simulink model "gm_sampleModel1884_1_sub"  (R2023a)
settings: Solver=VariableStepAuto  StartTime=0.0  StopTime=10.0  RelTol=1e-3
libraries: simulink x2
settings Model: Creator=user1  LastModifiedBy=user1
settings OptimizationCC: BlockReduction=off  ConditionallyExecuteInputs=off
settings DebuggingCC: InheritedTsInSrcMsg=none

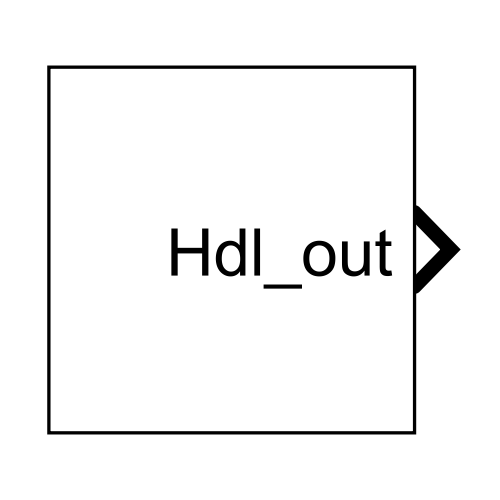
[thumbnail: Simulink's stored preview of the top-level diagram]
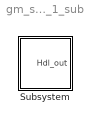
== system gm_sampleModel1884_1_sub ==
  Subsystem : Subsystem

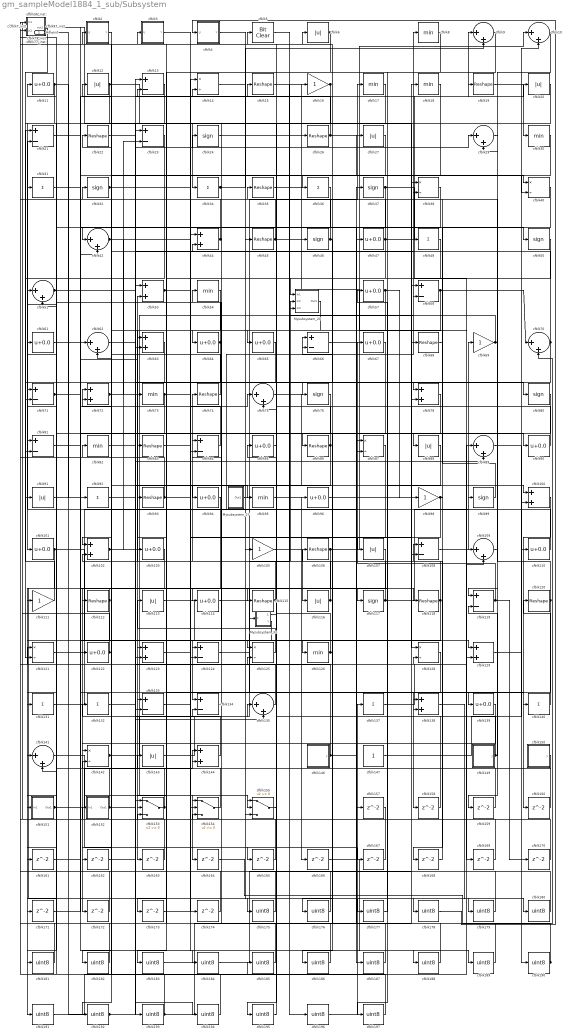
== system gm_sampleModel1884_1_sub/Subsystem ==
  Mysubsystem_20 : Subsystem
  Mysubsystem_27 : Subsystem
  Mysubsystem_33 : Subsystem
  cfblk{9..10,29,42,51,62,70,75,89,109,135,141} (12 alike) : Sum  Inputs=|++  OutDataTypeStr=uint8
  cfblk{44,53,63,72,78,100,102,123,129,138,144} (11 alike) : Sum  OutDataTypeStr=uint8
  cfblk{11,47,57,61,64..65,67,85,90,94,96,101,103,110,114,122,139} (17 alike) : Bias  Bias=0.0  SaturateOnIntegerOverflow=off
  cfblk{16,69,98,105,111} (5 alike) : Gain  OutDataTypeStr=uint8
  cfblk{15,19,22,26,35,45,68,74,83,86,93,106,112,115,118,120} (16 alike) : Reshape
  cfblk{6,12,20,27,88,91,107,113,116,143} (10 alike) : Abs  OutDataTypeStr=uint8  SaturateOnIntegerOverflow=off
  cfblk{13,21,23,58,66,71,81,84,108,119,124,133..134} (13 alike) : Sum  Inputs=+-  OutDataTypeStr=uint8
  cfblk{24,32,37,46,50,76,80,99,117} (9 alike) : Signum
  cfblk{14,38,40,87,121,125,128,142} (8 alike) : Product  Inputs=*/  OutDataTypeStr=uint8  RndMeth=Zero  SaturateOnIntegerOverflow=on
  cfblk{8,17..18,30,54,73,82,95,126} (9 alike) : MinMax  OutDataTypeStr=uint8
  cfblk127_inst : Subsystem
  cfblk{31,34,36,48,92,131..132,137,140} (9 alike) : Sum  Inputs=+  OutDataTypeStr=uint8
  cfblk136_inst : Subsystem
  cfblk146 : Subsystem  mask(Counter Limited){uplimit=double(7), tsamp=double(-1)}
      mask prompts: uplimit "Simulink:masks:UpperLimit_MP"; tsamp "Simulink:masks:SampleTime_MP"
      mask help: Simulink:masks:CounterLimited_MD
      mask init:
      | nbits = double(8);
      | tsamp = double(-1);
      | uplimit = double(7);
  cfblk147 : Constant  OutDataTypeStr=uint8  SampleTime=-1
  cfblk149 : Subsystem  mask(Counter Limited){uplimit=double(7), tsamp=double(-1)}
      mask prompts: uplimit "Simulink:masks:UpperLimit_MP"; tsamp "Simulink:masks:SampleTime_MP"
      mask help: Simulink:masks:CounterLimited_MD
      mask init:
      | nbits = double(8);
      | tsamp = double(-1);
      | uplimit = double(7);
  cfblk150 : Subsystem  mask(Counter Free-Running){NumBits=double(16), tsamp=double(-1)}
      mask prompts: NumBits "Simulink:masks:NumberOfBits_MP"; tsamp "Simulink:masks:SampleTime_MP"
      mask help: Simulink:masks:CounterFreeRunning_MD
  cfblk151 : Subsystem
  cfblk152 : Subsystem
  cfblk153 : Switch  OutDataTypeStr=uint8  SaturateOnIntegerOverflow=off  InputSameDT=off
  cfblk154 : Switch  OutDataTypeStr=uint8  SaturateOnIntegerOverflow=off  InputSameDT=off
  cfblk155 : Switch  OutDataTypeStr=uint8  SaturateOnIntegerOverflow=off  InputSameDT=off
  cfblk{157..174} (18 alike) : Delay  SampleTime=1
  cfblk{175..197} (23 alike) : DataTypeConversion  OutDataTypeStr=uint8  SaturateOnIntegerOverflow=off  RndMeth=Floor
  cfblk2 : Subsystem  mask(Detect Fall Nonpositive){vinit=double(0), InputProcessing=Elements as channels (sample based), OutDataTypeStr=uint8}
      mask prompts: vinit "Simulink:masks:InitialCondition_MP"; InputProcessing "Simulink:masks:InputProcessing_MP"; OutDataTypeStr "Simulink:masks:OutputDataType_MP"
      mask help: Simulink:masks:DetectFallNonpositive_MD
      mask init:
      | InputProcessing = 'Elements as channels (sample based)';
      | OutDataTypeStr = 'uint8';
      | vinit = double(0);
      mask TypeOptions InputProcessing: Simulink:masks:ColumnsAsChannelsFrameBased | Simulink:masks:ElementsAsChannelsSampleBased
      mask TypeOptions OutDataTypeStr: Simulink:masks:uint8 | Simulink:masks:boolean
      mask Display: fprintf('U <= 0\n&  NOT\nU/z <= 0')
  cfblk25_inst : Subsystem
  cfblk3 : Subsystem  mask(Detect Rise Positive){vinit=double(0), InputProcessing=Elements as channels (sample based), OutDataTypeStr=uint8}
      mask prompts: vinit "Simulink:masks:InitialCondition_MP"; InputProcessing "Simulink:masks:InputProcessing_MP"; OutDataTypeStr "Simulink:masks:OutputDataType_MP"
      mask help: Simulink:masks:DetectRisePositive_MD
      mask init:
      | InputProcessing = 'Elements as channels (sample based)';
      | OutDataTypeStr = 'uint8';
      | vinit = double(0);
      mask TypeOptions InputProcessing: Simulink:masks:ColumnsAsChannelsFrameBased | Simulink:masks:ElementsAsChannelsSampleBased
      mask TypeOptions OutDataTypeStr: Simulink:masks:uint8 | Simulink:masks:boolean
      mask Display: fprintf('U > 0\n&  NOT\nU/z > 0')
  cfblk4 : Subsystem  mask(Detect Rise Positive){vinit=double(0), InputProcessing=Elements as channels (sample based), OutDataTypeStr=uint8}
      mask prompts: vinit "Simulink:masks:InitialCondition_MP"; InputProcessing "Simulink:masks:InputProcessing_MP"; OutDataTypeStr "Simulink:masks:OutputDataType_MP"
      mask help: Simulink:masks:DetectRisePositive_MD
      mask init:
      | InputProcessing = 'Elements as channels (sample based)';
      | OutDataTypeStr = 'uint8';
      | vinit = double(0);
      mask TypeOptions InputProcessing: Simulink:masks:ColumnsAsChannelsFrameBased | Simulink:masks:ElementsAsChannelsSampleBased
      mask TypeOptions OutDataTypeStr: Simulink:masks:uint8 | Simulink:masks:boolean
      mask Display: fprintf('U > 0\n&  NOT\nU/z > 0')
  cfblk49_inst : Subsystem
  cfblk5 : simulink/Logic and Bit Operations/Bit Clear  iBit=0
      settings: LibrarySourceBlock=|
      | hdlsllib/Logic and Bit
      | Operations/Bit Clear
  cfblk52_inst : Subsystem
  cfblk56_inst : Subsystem
  cfblk77_inst : Subsystem
  cfblk79_inst : Subsystem
  cfblk7_inst : Subsystem
  cfblk97_inst : Subsystem
  Hdl_out : Outport  OutDataTypeStr=uint8  SampleTime=1
  wires:
  Mysubsystem_20/1(Out1) -> cfblk163/1
  Mysubsystem_27/1(Out1) -> cfblk100/1
  Mysubsystem_33/1(Out1) -> cfblk8/1
  Mysubsystem_33/2(Y) -> cfblk141/2
  cfblk10/1 -> cfblk29/2
  cfblk100/1 -> cfblk160/1
  cfblk101/1 -> cfblk178/1, cfblk129/1
  cfblk102/1 -> cfblk58/2, cfblk23/2, cfblk155/2
  cfblk103/1 -> cfblk191/1
  cfblk105/1 -> cfblk116/1
  cfblk106/1 -> cfblk10/1, cfblk172/1
  cfblk107/1 -> cfblk133/1
  cfblk108/1 -> cfblk69/1
  cfblk109/1 -> cfblk159/1
  cfblk11/1 -> cfblk101/1, cfblk92/1
  cfblk110/1 -> cfblk21/2
  cfblk111/1 -> cfblk21/1
  cfblk112/1 -> cfblk141/1, cfblk111/1
  cfblk113/1 -> cfblk126/1
  cfblk114/1 -> cfblk140/1
  cfblk115/1 -> cfblk53/2, cfblk22/1
  cfblk116/1 -> cfblk23/1, Mysubsystem_20/2(In2)
  cfblk117/1 -> cfblk99/1, cfblk74/1
  cfblk118/1 -> cfblk53/1, cfblk134/1, cfblk106/1
  cfblk119/1 -> cfblk67/1, cfblk170/1
  cfblk12/1 -> cfblk161/1, cfblk34/1
  cfblk120/1 -> cfblk35/1, cfblk158/1
  cfblk121/1 -> cfblk87/1
  cfblk122/1 -> cfblk62/2, cfblk49_inst/1(in1)
  cfblk123/1 -> cfblk174/1
  cfblk124/1 -> cfblk17/1
  cfblk125/1 -> cfblk113/1
  cfblk126/1 -> cfblk6/1, cfblk31/1
  cfblk127_inst/1(out1) -> cfblk128/1
  cfblk128/1 -> cfblk153/2
  cfblk129/1 -> cfblk10/2
  cfblk13/1 -> cfblk131/1
  cfblk131/1 -> cfblk16/1
  cfblk132/1 -> cfblk193/1
  cfblk133/1 -> cfblk27/1
  cfblk134/1 -> cfblk54/1
  cfblk135/1 -> cfblk77_inst/1(in1)
  cfblk136_inst/1(out1) -> cfblk105/1
  cfblk137/1 -> cfblk109/1
  cfblk138/1 -> cfblk180/1
  cfblk139/1 -> cfblk142/1
  cfblk14/1 -> cfblk45/1
  cfblk140/1 -> cfblk120/1
  cfblk141/1 -> cfblk165/1
  cfblk142/1 -> cfblk134/2, cfblk164/1
  cfblk143/1 -> cfblk46/1
  cfblk144/1 -> cfblk12/1
  cfblk146/1(y) -> cfblk47/1, cfblk82/1
  cfblk147/1 -> cfblk110/1
  cfblk149/1(y) -> cfblk119/2, cfblk14/2
  cfblk15/1 -> cfblk169/1
  cfblk150/1(y) -> cfblk142/2
  cfblk151/1(Out1) -> cfblk154/1, cfblk144/1, cfblk121/1
  cfblk152/1(Out1) -> cfblk135/1, cfblk127_inst/1(in1)
  cfblk153/1 -> cfblk72/1, cfblk32/1
  cfblk154/1 -> cfblk2/1(U)
  cfblk155/1 -> cfblk85/1
  cfblk157/1 -> cfblk153/3
  cfblk158/1 -> cfblk44/2
  cfblk159/1 -> cfblk71/1
  cfblk16/1 -> cfblk65/1, cfblk121/2
  cfblk160/1 -> cfblk84/1
  cfblk161/1 -> cfblk42/2
  cfblk162/1 -> cfblk128/2
  cfblk163/1 -> cfblk136_inst/2(in2)
  cfblk164/1 -> cfblk70/2
  cfblk165/1 -> cfblk52_inst/1(in1)
  cfblk166/1 -> cfblk189/1
  cfblk167/1 -> cfblk153/1
  cfblk168/1 -> cfblk108/1
  cfblk169/1 -> cfblk58/1
  cfblk17/1 -> cfblk114/1
  cfblk170/1 -> cfblk102/2
  cfblk171/1 -> cfblk63/1
  cfblk172/1 -> cfblk51/1
  cfblk173/1 -> cfblk125/2
  cfblk174/1 -> cfblk81/1
  cfblk175/1 -> cfblk11/1
  cfblk176/1 -> cfblk3/1(U)
  cfblk177/1 -> cfblk57/1
  cfblk178/1 -> cfblk4/1(U)
  cfblk179/1 -> cfblk75/2
  cfblk18/1 -> cfblk182/1
  cfblk180/1 -> cfblk25_inst/1(in1)
  cfblk181/1 -> cfblk25_inst/2(in2)
  cfblk182/1 -> cfblk79_inst/1(in1)
  cfblk183/1 -> cfblk18/1
  cfblk184/1 -> cfblk68/1
  cfblk185/1 -> cfblk7_inst/1(in1)
  cfblk186/1 -> cfblk7_inst/2(in2)
  cfblk187/1 -> cfblk143/1
  cfblk188/1 -> cfblk66/1
  cfblk189/1 -> cfblk66/2
  cfblk19/1 -> cfblk30/1
  cfblk190/1 -> cfblk72/2, cfblk154/3, cfblk144/2, cfblk152/1(In1)
  cfblk191/1 -> cfblk89/1
  cfblk192/1 -> cfblk89/2, Hdl_out/1
  cfblk193/1 -> cfblk79_inst/2(in2), cfblk37/1, cfblk185/1
  cfblk194/1 -> cfblk132/1
  cfblk195/1 -> cfblk5/1
  cfblk196/1 -> cfblk137/1
  cfblk197/1 -> cfblk61/1
  cfblk2/1(Y) -> cfblk162/1
  cfblk20/1 -> cfblk63/2
  cfblk21/1 -> cfblk40/1
  cfblk22/1 -> cfblk95/1
  cfblk23/1 -> cfblk71/2
  cfblk24/1 -> cfblk26/1
  cfblk25_inst/1(out1) -> cfblk179/1
  cfblk26/1 -> cfblk15/1, cfblk40/2
  cfblk27/1 -> cfblk36/1
  cfblk29/1 -> cfblk139/1
  cfblk3/1(Y) -> cfblk175/1
  cfblk30/1 -> cfblk42/1
  cfblk31/1 -> cfblk86/1
  cfblk32/1 -> cfblk155/1, cfblk108/2
  cfblk34/1 -> cfblk9/2, cfblk155/3, cfblk124/1
  cfblk35/1 -> cfblk157/1
  cfblk36/1 -> Mysubsystem_33/1(In1)
  cfblk37/1 -> cfblk109/2, cfblk87/2
  cfblk38/1 -> cfblk171/1
  cfblk4/1(Y) -> cfblk177/1
  cfblk40/1 -> cfblk78/1
  cfblk42/1 -> cfblk80/1, cfblk73/1
  cfblk44/1 -> cfblk64/1, cfblk136_inst/1(in1)
  cfblk45/1 -> cfblk96/1, cfblk127_inst/2(in2)
  cfblk46/1 -> cfblk76/1, cfblk49_inst/2(in2)
  cfblk47/1 -> cfblk9/1, cfblk123/1, cfblk14/1
  cfblk48/1 -> cfblk94/1
  cfblk49_inst/1(out1) -> cfblk50/1, cfblk118/1
  cfblk5/1 -> cfblk196/1
  cfblk50/1 -> Mysubsystem_20/1(In1)
  cfblk51/1 -> cfblk19/1, cfblk135/2
  cfblk52_inst/1(out1) -> cfblk84/2
  cfblk53/1 -> cfblk129/2, cfblk167/1
  cfblk54/1 -> cfblk112/1
  cfblk56_inst/1(out1) -> cfblk91/1
  cfblk57/1 -> cfblk115/1, cfblk98/1
  cfblk58/1 -> cfblk93/1, cfblk70/1
  cfblk6/1 -> cfblk77_inst/2(in2), cfblk124/2
  cfblk61/1 -> cfblk62/1
  cfblk62/1 -> cfblk20/1
  cfblk63/1 -> cfblk81/2
  cfblk64/1 -> cfblk97_inst/2(in2), cfblk192/1
  cfblk65/1 -> cfblk173/1
  cfblk66/1 -> cfblk187/1
  cfblk67/1 -> cfblk176/1
  cfblk68/1 -> cfblk138/2
  cfblk69/1 -> cfblk119/1, Mysubsystem_20/3(In3)
  cfblk7_inst/1(out1) -> cfblk184/1
  cfblk70/1 -> cfblk52_inst/2(in2), cfblk123/2
  cfblk71/1 -> cfblk51/2, cfblk13/2
  cfblk72/1 -> cfblk78/2, cfblk194/1
  cfblk73/1 -> cfblk83/1, cfblk188/1
  cfblk74/1 -> cfblk56_inst/2(in2)
  cfblk75/1 -> cfblk100/2
  cfblk76/1 -> cfblk103/1
  cfblk77_inst/1(out1) -> cfblk88/1
  cfblk78/1 -> cfblk151/1(In1)
  cfblk79_inst/1(out1) -> cfblk138/1
  cfblk8/1 -> cfblk197/1
  cfblk80/1 -> cfblk181/1
  cfblk81/1 -> cfblk125/1
  cfblk82/1 -> cfblk48/1
  cfblk83/1 -> cfblk90/1
  cfblk84/1 -> cfblk44/1
  cfblk85/1 -> cfblk195/1
  cfblk86/1 -> cfblk13/1, cfblk102/1
  cfblk87/1 -> cfblk107/1
  cfblk88/1 -> cfblk117/1
  cfblk89/1 -> cfblk190/1
  cfblk9/1 -> cfblk183/1
  cfblk90/1 -> cfblk56_inst/1(in1)
  cfblk91/1 -> cfblk75/1
  cfblk92/1 -> cfblk24/1
  cfblk93/1 -> cfblk97_inst/1(in1), cfblk29/1
  cfblk94/1 -> cfblk122/1
  cfblk95/1 -> cfblk166/1
  cfblk96/1 -> cfblk38/1
  cfblk97_inst/1(out1) -> cfblk133/2
  cfblk98/1 -> cfblk186/1, cfblk154/2, cfblk168/1
  cfblk99/1 -> cfblk38/2

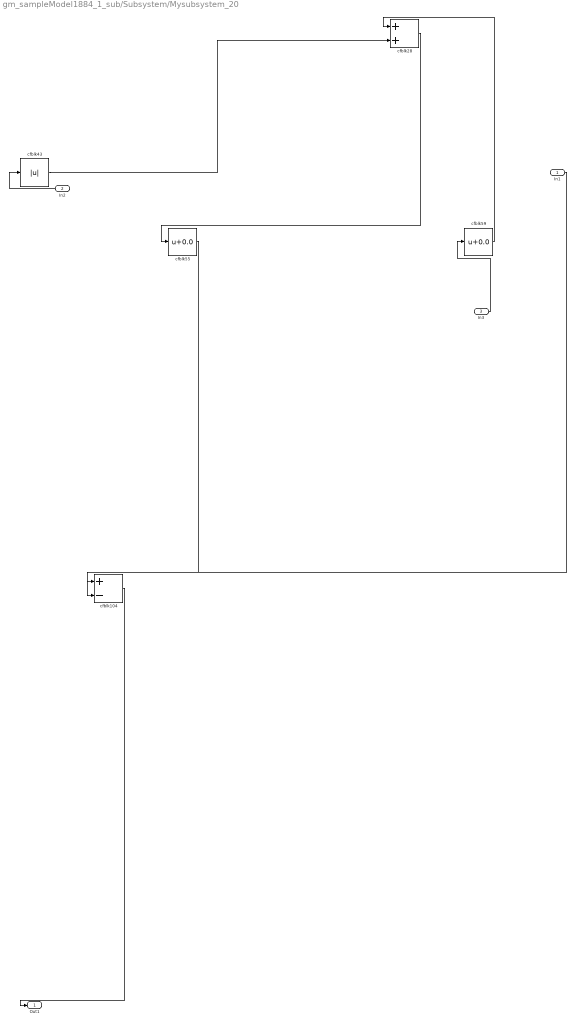
== system gm_sampleModel1884_1_sub/Subsystem/Mysubsystem_20 ==
  In1 : Inport  OutDataTypeStr=uint8  PortDimensions=1  SampleTime=1
  In2 : Inport  Port=2  OutDataTypeStr=uint8  PortDimensions=1  SampleTime=1
  In3 : Inport  Port=3  OutDataTypeStr=uint8  PortDimensions=1  SampleTime=1
  cfblk104 : Sum  Inputs=+-
  cfblk28 : Sum
  cfblk43 : Abs  SaturateOnIntegerOverflow=off
  cfblk55 : Bias  Bias=0.0  SaturateOnIntegerOverflow=off
  cfblk59 : Bias  Bias=0.0  SaturateOnIntegerOverflow=off
  Out1 : Outport  SampleTime=1
  wires:
  In1/1 -> cfblk104/2
  In2/1 -> cfblk43/1
  In3/1 -> cfblk59/1
  cfblk104/1 -> Out1/1
  cfblk28/1 -> cfblk55/1
  cfblk43/1 -> cfblk28/2
  cfblk55/1 -> cfblk104/1
  cfblk59/1 -> cfblk28/1

== system gm_sampleModel1884_1_sub/Subsystem/Mysubsystem_27 ==
  cfblk148 : Ground
  cfblk41 : Sum  Inputs=+
  Out1 : Outport  SampleTime=1
  wires:
  cfblk148/1 -> cfblk41/1
  cfblk41/1 -> Out1/1

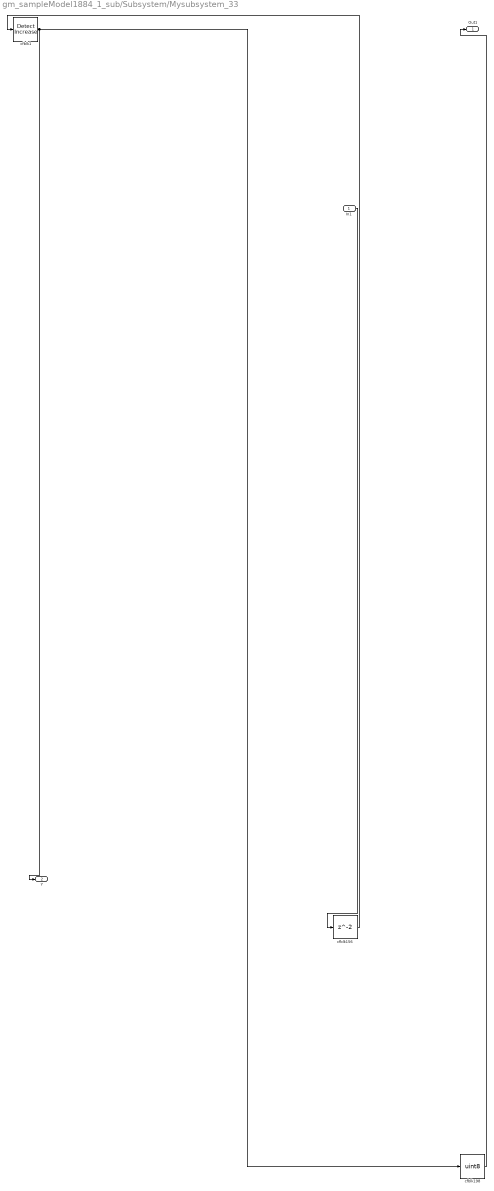
== system gm_sampleModel1884_1_sub/Subsystem/Mysubsystem_33 ==
  In1 : Inport  OutDataTypeStr=uint8  PortDimensions=1  SampleTime=1
  cfblk1 : simulink/Logic and Bit Operations/Detect Increase  vinit=0.0  OutDataTypeStr=boolean
      settings: LibrarySourceBlock=|
      | hdlsllib/Logic and Bit
      | Operations/Detect
      | Increase
  cfblk156 : Delay  SampleTime=1
  cfblk198 : DataTypeConversion  OutDataTypeStr=uint8  SaturateOnIntegerOverflow=off  RndMeth=Floor
  Out1 : Outport  SampleTime=1
  Y : Outport  Port=2  SampleTime=1
  wires:
  In1/1 -> cfblk156/1
  cfblk1/1 -> cfblk198/1, Y/1
  cfblk156/1 -> cfblk1/1
  cfblk198/1 -> Out1/1

== system gm_sampleModel1884_1_sub/Subsystem/cfblk127_inst ==
  in1 : Inport  OutDataTypeStr=uint8  SampleTime=1
  in2 : Inport  Port=2  OutDataTypeStr=uint8  SampleTime=1
  mul_cfblk127_dotp_mulcomp : Product  Inputs=**  OutDataTypeStr=uint8  SampleTime=1
  out1 : Outport  OutDataTypeStr=uint8  SampleTime=1
  wires:
  in1/1 -> mul_cfblk127_dotp_mulcomp/1
  in2/1 -> mul_cfblk127_dotp_mulcomp/2
  mul_cfblk127_dotp_mulcomp/1 -> out1/1

== system gm_sampleModel1884_1_sub/Subsystem/cfblk136_inst ==
  in1 : Inport  OutDataTypeStr=uint8  SampleTime=1
  in2 : Inport  Port=2  OutDataTypeStr=uint8  SampleTime=1
  mul_cfblk136_dotp_mulcomp : Product  Inputs=**  OutDataTypeStr=uint8  SampleTime=1
  out1 : Outport  OutDataTypeStr=uint8  SampleTime=1
  wires:
  in1/1 -> mul_cfblk136_dotp_mulcomp/1
  in2/1 -> mul_cfblk136_dotp_mulcomp/2
  mul_cfblk136_dotp_mulcomp/1 -> out1/1

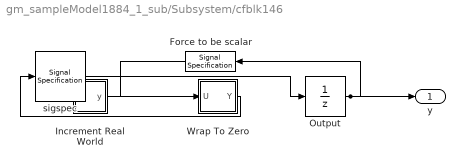
== system gm_sampleModel1884_1_sub/Subsystem/cfblk146 ==
  Force to be scalar : SignalSpecification  DisableCoverage=on  Dimensions=1
  Increment Real World : Subsystem  mask(Real World Value Increment){}
      mask help: Simulink:masks:RealWorldValueIncrement_MD
      mask Display: disp('V++')
  Output : UnitDelay  InitialCondition=0.0  SampleTime=tsamp  HasFrameUpgradeWarning=on
  Wrap To Zero : Subsystem  mask(Wrap To Zero){Threshold=double(7)}
      mask prompts: Threshold "Simulink:masks:Threshold_MP"
      mask help: Simulink:masks:WrapToZero_MD
  sigspec : SignalSpecification  OutDataTypeStr=uint8  Dimensions=1
  y : Outport  SampleTime=1
  wires:
  Force to be scalar/1 -> Increment Real World/1(u)
  Increment Real World/1(y) -> Wrap To Zero/1(U)
  Output/1 -> Force to be scalar/1, y/1
  Wrap To Zero/1(Y) -> sigspec/1
  sigspec/1 -> Output/1

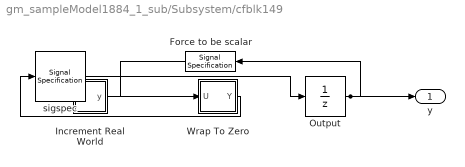
== system gm_sampleModel1884_1_sub/Subsystem/cfblk149 ==
  Force to be scalar : SignalSpecification  DisableCoverage=on  Dimensions=1
  Increment Real World : Subsystem  mask(Real World Value Increment){}
      mask help: Simulink:masks:RealWorldValueIncrement_MD
      mask Display: disp('V++')
  Output : UnitDelay  InitialCondition=0.0  SampleTime=tsamp  HasFrameUpgradeWarning=on
  Wrap To Zero : Subsystem  mask(Wrap To Zero){Threshold=double(7)}
      mask prompts: Threshold "Simulink:masks:Threshold_MP"
      mask help: Simulink:masks:WrapToZero_MD
  sigspec : SignalSpecification  OutDataTypeStr=uint8  Dimensions=1
  y : Outport  SampleTime=1
  wires:
  Force to be scalar/1 -> Increment Real World/1(u)
  Increment Real World/1(y) -> Wrap To Zero/1(U)
  Output/1 -> Force to be scalar/1, y/1
  Wrap To Zero/1(Y) -> sigspec/1
  sigspec/1 -> Output/1

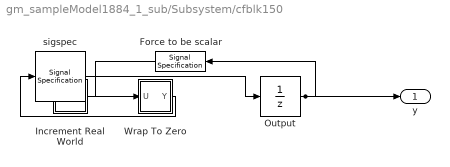
== system gm_sampleModel1884_1_sub/Subsystem/cfblk150 ==
  Force to be scalar : SignalSpecification  DisableCoverage=on  Dimensions=1
  Increment Real World : Subsystem  mask(Real World Value Increment){}
      mask help: Simulink:masks:RealWorldValueIncrement_MD
      mask Display: disp('V++')
  Output : UnitDelay  InitialCondition=0.0  SampleTime=tsamp  HasFrameUpgradeWarning=on
  Wrap To Zero : Subsystem  mask(Wrap To Zero){Threshold=double(65535)}
      mask prompts: Threshold "Simulink:masks:Threshold_MP"
      mask help: Simulink:masks:WrapToZero_MD
  sigspec : SignalSpecification  OutDataTypeStr=uint16  Dimensions=1
  y : Outport  SampleTime=1
  wires:
  Force to be scalar/1 -> Increment Real World/1(u)
  Increment Real World/1(y) -> Wrap To Zero/1(U)
  Output/1 -> Force to be scalar/1, y/1
  Wrap To Zero/1(Y) -> sigspec/1
  sigspec/1 -> Output/1

== system gm_sampleModel1884_1_sub/Subsystem/cfblk151 ==
  In1 : Inport  OutDataTypeStr=uint8  PortDimensions=1  SampleTime=1
  Out1 : Outport  SampleTime=1
  wires:
  In1/1 -> Out1/1

== system gm_sampleModel1884_1_sub/Subsystem/cfblk152 ==
  In1 : Inport  OutDataTypeStr=uint8  PortDimensions=1  SampleTime=1
  Out1 : Outport  SampleTime=1
  wires:
  In1/1 -> Out1/1

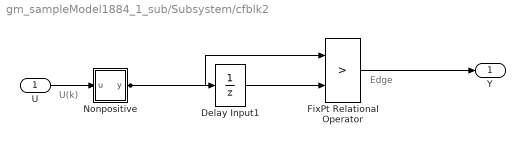
== system gm_sampleModel1884_1_sub/Subsystem/cfblk2 ==
  note: U(k)
  note: Edge
  U : Inport  OutDataTypeStr=uint8  SampleTime=1
  Delay Input1 : UnitDelay  Description=Store in Global RAM  DisableCoverage=on  InitialCondition=vinit  SampleTime=-1  HasFrameUpgradeWarning=on
  FixPt Relational Operator : RelationalOperator  Operator=>  OutDataTypeStr=fixdt(0, 8)  ZeroCross=off  InputSameDT=off
  Nonpositive : Subsystem  mask(Compare To Zero){relop=<=, OutDataTypeStr=boolean, ZeroCross=off}
      mask prompts: relop "Simulink:masks:Operator_MP"; OutDataTypeStr "Simulink:masks:OutputDataType_MP"; ZeroCross "Simulink:masks:EnableZerocrossingDetection_MP"
      mask help: Simulink:masks:CompareToZero_MD
      mask init:
      | OutDataTypeStr = 'boolean';
      | ZeroCross = 'off';
      | blkName = 'sampleModel1884_1_sub/Subsystem/cfblk2/Nonpositive';
      | relop = '<=';
      | setValue = 'boolean';
      mask TypeOptions relop: == | ~= | < | <= | >= | >
      mask TypeOptions OutDataTypeStr: Simulink:masks:uint8 | Simulink:masks:boolean
      mask Callback ZeroCross: sl('zeroCrossEnable', gcbh);
      mask Display: disp([relop,' 0'])
  Y : Outport  SampleTime=1
  wires:
  U/1 -> Nonpositive/1(u)
  Delay Input1/1 -> FixPt Relational Operator/2
  FixPt Relational Operator/1 -> Y/1
  Nonpositive/1(y) -> FixPt Relational Operator/1, Delay Input1/1

== system gm_sampleModel1884_1_sub/Subsystem/cfblk25_inst ==
  in1 : Inport  OutDataTypeStr=uint8  SampleTime=1
  in2 : Inport  Port=2  OutDataTypeStr=uint8  SampleTime=1
  mul_cfblk25_dotp_mulcomp : Product  Inputs=**  OutDataTypeStr=uint8  SampleTime=1
  out1 : Outport  OutDataTypeStr=uint8  SampleTime=1
  wires:
  in1/1 -> mul_cfblk25_dotp_mulcomp/1
  in2/1 -> mul_cfblk25_dotp_mulcomp/2
  mul_cfblk25_dotp_mulcomp/1 -> out1/1

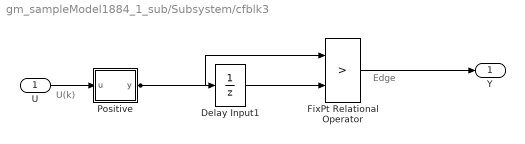
== system gm_sampleModel1884_1_sub/Subsystem/cfblk3 ==
  note: U(k)
  note: Edge
  U : Inport  OutDataTypeStr=uint8  SampleTime=1
  Delay Input1 : UnitDelay  Description=Store in Global RAM  DisableCoverage=on  InitialCondition=vinit  SampleTime=-1  HasFrameUpgradeWarning=on
  FixPt Relational Operator : RelationalOperator  Operator=>  OutDataTypeStr=fixdt(0, 8)  ZeroCross=off  InputSameDT=off
  Positive : Subsystem  mask(Compare To Zero){relop=>, OutDataTypeStr=boolean, ZeroCross=off}
      mask prompts: relop "Simulink:masks:Operator_MP"; OutDataTypeStr "Simulink:masks:OutputDataType_MP"; ZeroCross "Simulink:masks:EnableZerocrossingDetection_MP"
      mask help: Simulink:masks:CompareToZero_MD
      mask init:
      | OutDataTypeStr = 'boolean';
      | ZeroCross = 'off';
      | blkName = 'sampleModel1884_1_sub/Subsystem/cfblk3/Positive';
      | relop = '>';
      | setValue = 'boolean';
      mask TypeOptions relop: == | ~= | < | <= | >= | >
      mask TypeOptions OutDataTypeStr: Simulink:masks:uint8 | Simulink:masks:boolean
      mask Callback ZeroCross: sl('zeroCrossEnable', gcbh);
      mask Display: disp([relop,' 0'])
  Y : Outport  SampleTime=1
  wires:
  U/1 -> Positive/1(u)
  Delay Input1/1 -> FixPt Relational Operator/2
  FixPt Relational Operator/1 -> Y/1
  Positive/1(y) -> FixPt Relational Operator/1, Delay Input1/1

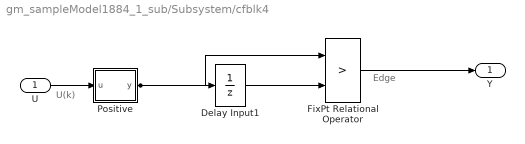
== system gm_sampleModel1884_1_sub/Subsystem/cfblk4 ==
  note: U(k)
  note: Edge
  U : Inport  OutDataTypeStr=uint8  SampleTime=1
  Delay Input1 : UnitDelay  Description=Store in Global RAM  DisableCoverage=on  InitialCondition=vinit  SampleTime=-1  HasFrameUpgradeWarning=on
  FixPt Relational Operator : RelationalOperator  Operator=>  OutDataTypeStr=fixdt(0, 8)  ZeroCross=off  InputSameDT=off
  Positive : Subsystem  mask(Compare To Zero){relop=>, OutDataTypeStr=boolean, ZeroCross=off}
      mask prompts: relop "Simulink:masks:Operator_MP"; OutDataTypeStr "Simulink:masks:OutputDataType_MP"; ZeroCross "Simulink:masks:EnableZerocrossingDetection_MP"
      mask help: Simulink:masks:CompareToZero_MD
      mask init:
      | OutDataTypeStr = 'boolean';
      | ZeroCross = 'off';
      | blkName = 'sampleModel1884_1_sub/Subsystem/cfblk4/Positive';
      | relop = '>';
      | setValue = 'boolean';
      mask TypeOptions relop: == | ~= | < | <= | >= | >
      mask TypeOptions OutDataTypeStr: Simulink:masks:uint8 | Simulink:masks:boolean
      mask Callback ZeroCross: sl('zeroCrossEnable', gcbh);
      mask Display: disp([relop,' 0'])
  Y : Outport  SampleTime=1
  wires:
  U/1 -> Positive/1(u)
  Delay Input1/1 -> FixPt Relational Operator/2
  FixPt Relational Operator/1 -> Y/1
  Positive/1(y) -> FixPt Relational Operator/1, Delay Input1/1

== system gm_sampleModel1884_1_sub/Subsystem/cfblk49_inst ==
  in1 : Inport  OutDataTypeStr=uint8  SampleTime=1
  in2 : Inport  Port=2  OutDataTypeStr=uint8  SampleTime=1
  mul_cfblk49_dotp_mulcomp : Product  Inputs=**  OutDataTypeStr=uint8  SampleTime=1
  out1 : Outport  OutDataTypeStr=uint8  SampleTime=1
  wires:
  in1/1 -> mul_cfblk49_dotp_mulcomp/1
  in2/1 -> mul_cfblk49_dotp_mulcomp/2
  mul_cfblk49_dotp_mulcomp/1 -> out1/1

== system gm_sampleModel1884_1_sub/Subsystem/cfblk52_inst ==
  in1 : Inport  OutDataTypeStr=uint8  SampleTime=1
  in2 : Inport  Port=2  OutDataTypeStr=uint8  SampleTime=1
  mul_cfblk52_dotp_mulcomp : Product  Inputs=**  OutDataTypeStr=uint8  SampleTime=1
  out1 : Outport  OutDataTypeStr=uint8  SampleTime=1
  wires:
  in1/1 -> mul_cfblk52_dotp_mulcomp/1
  in2/1 -> mul_cfblk52_dotp_mulcomp/2
  mul_cfblk52_dotp_mulcomp/1 -> out1/1

== system gm_sampleModel1884_1_sub/Subsystem/cfblk56_inst ==
  in1 : Inport  OutDataTypeStr=uint8  SampleTime=1
  in2 : Inport  Port=2  OutDataTypeStr=uint8  SampleTime=1
  mul_cfblk56_dotp_mulcomp : Product  Inputs=**  OutDataTypeStr=uint8  SampleTime=1
  out1 : Outport  OutDataTypeStr=uint8  SampleTime=1
  wires:
  in1/1 -> mul_cfblk56_dotp_mulcomp/1
  in2/1 -> mul_cfblk56_dotp_mulcomp/2
  mul_cfblk56_dotp_mulcomp/1 -> out1/1

== system gm_sampleModel1884_1_sub/Subsystem/cfblk77_inst ==
  in1 : Inport  OutDataTypeStr=uint8  SampleTime=1
  in2 : Inport  Port=2  OutDataTypeStr=uint8  SampleTime=1
  mul_cfblk77_dotp_mulcomp : Product  Inputs=**  OutDataTypeStr=uint8  SampleTime=1
  out1 : Outport  OutDataTypeStr=uint8  SampleTime=1
  wires:
  in1/1 -> mul_cfblk77_dotp_mulcomp/1
  in2/1 -> mul_cfblk77_dotp_mulcomp/2
  mul_cfblk77_dotp_mulcomp/1 -> out1/1

== system gm_sampleModel1884_1_sub/Subsystem/cfblk79_inst ==
  in1 : Inport  OutDataTypeStr=uint8  SampleTime=1
  in2 : Inport  Port=2  OutDataTypeStr=uint8  SampleTime=1
  mul_cfblk79_dotp_mulcomp : Product  Inputs=**  OutDataTypeStr=uint8  SampleTime=1
  out1 : Outport  OutDataTypeStr=uint8  SampleTime=1
  wires:
  in1/1 -> mul_cfblk79_dotp_mulcomp/1
  in2/1 -> mul_cfblk79_dotp_mulcomp/2
  mul_cfblk79_dotp_mulcomp/1 -> out1/1

== system gm_sampleModel1884_1_sub/Subsystem/cfblk7_inst ==
  in1 : Inport  OutDataTypeStr=uint8  SampleTime=1
  in2 : Inport  Port=2  OutDataTypeStr=uint8  SampleTime=1
  mul_cfblk7_dotp_mulcomp : Product  Inputs=**  OutDataTypeStr=uint8  SampleTime=1
  out1 : Outport  OutDataTypeStr=uint8  SampleTime=1
  wires:
  in1/1 -> mul_cfblk7_dotp_mulcomp/1
  in2/1 -> mul_cfblk7_dotp_mulcomp/2
  mul_cfblk7_dotp_mulcomp/1 -> out1/1

== system gm_sampleModel1884_1_sub/Subsystem/cfblk97_inst ==
  in1 : Inport  OutDataTypeStr=uint8  SampleTime=1
  in2 : Inport  Port=2  OutDataTypeStr=uint8  SampleTime=1
  mul_cfblk97_dotp_mulcomp : Product  Inputs=**  OutDataTypeStr=uint8  SampleTime=1
  out1 : Outport  OutDataTypeStr=uint8  SampleTime=1
  wires:
  in1/1 -> mul_cfblk97_dotp_mulcomp/1
  in2/1 -> mul_cfblk97_dotp_mulcomp/2
  mul_cfblk97_dotp_mulcomp/1 -> out1/1

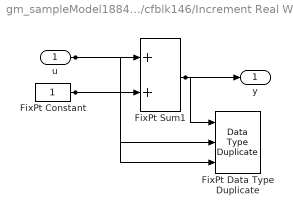
== system gm_sampleModel1884_1_sub/Subsystem/cfblk146/Increment Real World ==
  u : Inport  OutDataTypeStr=uint8  SampleTime=1
  FixPt Constant : Constant  DisableCoverage=on  OutDataTypeStr=Inherit: Inherit via back propagation  SampleTime=-1
  FixPt Data Type Duplicate : DataTypeDuplicate  DisableCoverage=on  NumInputPorts=3
  FixPt Sum1 : Sum  InputSameDT=on  OutDataTypeStr=Inherit: Inherit via back propagation  LockScale=on
  y : Outport  SampleTime=1
  wires:
  u/1 -> FixPt Sum1/1, FixPt Data Type Duplicate/2
  FixPt Constant/1 -> FixPt Sum1/2, FixPt Data Type Duplicate/3
  FixPt Sum1/1 -> FixPt Data Type Duplicate/1, y/1

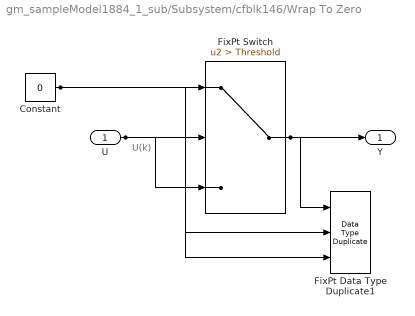
== system gm_sampleModel1884_1_sub/Subsystem/cfblk146/Wrap To Zero ==
  note: U(k)
  U : Inport  OutDataTypeStr=uint8  SampleTime=1
  Constant : Constant  DisableCoverage=on  Value=0  OutDataTypeStr=Inherit: Inherit via back propagation  SampleTime=-1
  FixPt Data Type Duplicate1 : DataTypeDuplicate  DisableCoverage=on  NumInputPorts=3
  FixPt Switch : Switch  Criteria=u2 > Threshold  Threshold=Threshold  OutDataTypeStr=Inherit: Inherit via back propagation  ZeroCross=off  SaturateOnIntegerOverflow=off  InputSameDT=off
  Y : Outport  SampleTime=1
  wires:
  U/1 -> FixPt Switch/3, FixPt Switch/2, FixPt Data Type Duplicate1/2
  Constant/1 -> FixPt Switch/1, FixPt Data Type Duplicate1/3
  FixPt Switch/1 -> FixPt Data Type Duplicate1/1, Y/1

== system gm_sampleModel1884_1_sub/Subsystem/cfblk149/Increment Real World ==
  u : Inport  OutDataTypeStr=uint8  SampleTime=1
  FixPt Constant : Constant  DisableCoverage=on  OutDataTypeStr=Inherit: Inherit via back propagation  SampleTime=-1
  FixPt Data Type Duplicate : DataTypeDuplicate  DisableCoverage=on  NumInputPorts=3
  FixPt Sum1 : Sum  InputSameDT=on  OutDataTypeStr=Inherit: Inherit via back propagation  LockScale=on
  y : Outport  SampleTime=1
  wires:
  u/1 -> FixPt Sum1/1, FixPt Data Type Duplicate/2
  FixPt Constant/1 -> FixPt Sum1/2, FixPt Data Type Duplicate/3
  FixPt Sum1/1 -> FixPt Data Type Duplicate/1, y/1

== system gm_sampleModel1884_1_sub/Subsystem/cfblk149/Wrap To Zero ==
  note: U(k)
  U : Inport  OutDataTypeStr=uint8  SampleTime=1
  Constant : Constant  DisableCoverage=on  Value=0  OutDataTypeStr=Inherit: Inherit via back propagation  SampleTime=-1
  FixPt Data Type Duplicate1 : DataTypeDuplicate  DisableCoverage=on  NumInputPorts=3
  FixPt Switch : Switch  Criteria=u2 > Threshold  Threshold=Threshold  OutDataTypeStr=Inherit: Inherit via back propagation  ZeroCross=off  SaturateOnIntegerOverflow=off  InputSameDT=off
  Y : Outport  SampleTime=1
  wires:
  U/1 -> FixPt Switch/3, FixPt Switch/2, FixPt Data Type Duplicate1/2
  Constant/1 -> FixPt Switch/1, FixPt Data Type Duplicate1/3
  FixPt Switch/1 -> FixPt Data Type Duplicate1/1, Y/1

== system gm_sampleModel1884_1_sub/Subsystem/cfblk150/Increment Real World ==
  u : Inport  OutDataTypeStr=uint16  SampleTime=1
  FixPt Constant : Constant  DisableCoverage=on  OutDataTypeStr=Inherit: Inherit via back propagation  SampleTime=-1
  FixPt Data Type Duplicate : DataTypeDuplicate  DisableCoverage=on  NumInputPorts=3
  FixPt Sum1 : Sum  InputSameDT=on  OutDataTypeStr=Inherit: Inherit via back propagation  LockScale=on
  y : Outport  SampleTime=1
  wires:
  u/1 -> FixPt Sum1/1, FixPt Data Type Duplicate/2
  FixPt Constant/1 -> FixPt Sum1/2, FixPt Data Type Duplicate/3
  FixPt Sum1/1 -> FixPt Data Type Duplicate/1, y/1

== system gm_sampleModel1884_1_sub/Subsystem/cfblk150/Wrap To Zero ==
  note: U(k)
  U : Inport  OutDataTypeStr=uint16  SampleTime=1
  Constant : Constant  DisableCoverage=on  Value=0  OutDataTypeStr=Inherit: Inherit via back propagation  SampleTime=-1
  FixPt Data Type Duplicate1 : DataTypeDuplicate  DisableCoverage=on  NumInputPorts=3
  FixPt Switch : Switch  Criteria=u2 > Threshold  Threshold=Threshold  OutDataTypeStr=Inherit: Inherit via back propagation  ZeroCross=off  SaturateOnIntegerOverflow=off  InputSameDT=off
  Y : Outport  SampleTime=1
  wires:
  U/1 -> FixPt Switch/3, FixPt Switch/2, FixPt Data Type Duplicate1/2
  Constant/1 -> FixPt Switch/1, FixPt Data Type Duplicate1/3
  FixPt Switch/1 -> FixPt Data Type Duplicate1/1, Y/1

== system gm_sampleModel1884_1_sub/Subsystem/cfblk2/Nonpositive ==
  u : Inport  OutDataTypeStr=uint8  SampleTime=1
  Compare : RelationalOperator  Operator=<=  OutDataTypeStr=boolean  ZeroCross=off
  Constant : Constant  DisableCoverage=on  Value=0  OutDataTypeStr=Inherit: Inherit via back propagation  SampleTime=-1  PreserveConstantTs=on
  y : Outport  SampleTime=1
  wires:
  u/1 -> Compare/1
  Compare/1 -> y/1
  Constant/1 -> Compare/2

== system gm_sampleModel1884_1_sub/Subsystem/cfblk3/Positive ==
  u : Inport  OutDataTypeStr=uint8  SampleTime=1
  Compare : RelationalOperator  Operator=>  OutDataTypeStr=boolean  ZeroCross=off
  Constant : Constant  DisableCoverage=on  Value=0  OutDataTypeStr=Inherit: Inherit via back propagation  SampleTime=-1  PreserveConstantTs=on
  y : Outport  SampleTime=1
  wires:
  u/1 -> Compare/1
  Compare/1 -> y/1
  Constant/1 -> Compare/2

== system gm_sampleModel1884_1_sub/Subsystem/cfblk4/Positive ==
  u : Inport  OutDataTypeStr=uint8  SampleTime=1
  Compare : RelationalOperator  Operator=>  OutDataTypeStr=boolean  ZeroCross=off
  Constant : Constant  DisableCoverage=on  Value=0  OutDataTypeStr=Inherit: Inherit via back propagation  SampleTime=-1  PreserveConstantTs=on
  y : Outport  SampleTime=1
  wires:
  u/1 -> Compare/1
  Compare/1 -> y/1
  Constant/1 -> Compare/2
